simulink model "GA_NoSin_Lin"  (R2017a)
settings: Solver=FixedStepAuto  StartTime=0.0  StopTime=4*pi  MaxStep=1e-4  RelTol=1e-6
libraries: powerlib x6, powerlib_meascontrol x3
settings Model: Creator=pagilm  LastModifiedBy=pagilm

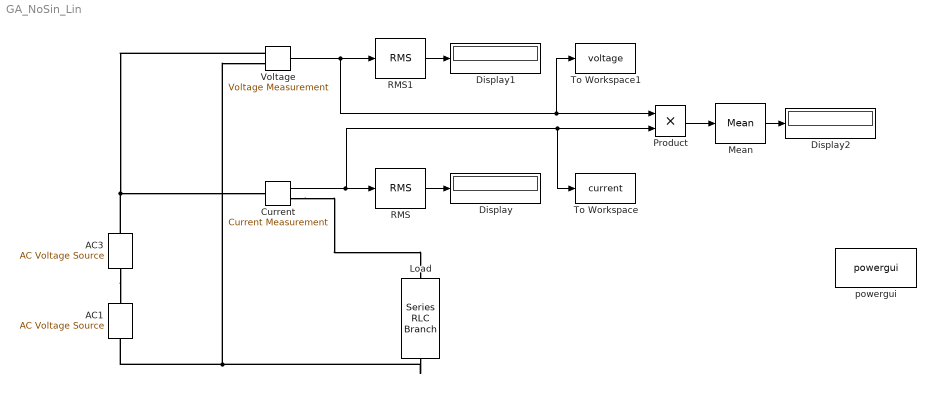
== system GA_NoSin_Lin ==
  AC1 : powerlib/Electrical Sources/AC Voltage Source  Amplitude=200*sqrt(2)  Phase=0  Frequency=1/2/pi  SampleTime=0  Measurements=None  BusType=swing  Pref=10e3  Qref=0  Qmin=-inf  Qmax=+inf
  AC3 : powerlib/Electrical Sources/AC Voltage Source  Amplitude=200*sqrt(2)  Phase=0  Frequency=3/2/pi  SampleTime=0  Measurements=None  BusType=swing  Pref=10e3  Qref=0  Qmin=-inf  Qmax=+inf
  "Current " : powerlib/Measurements/Current Measurement  PhasorSimulation=off  OutputType=Complex  PSBequivalent=0
  Display : Display
  Display1 : Display
  Display2 : Display
  Load : powerlib/Elements/Series RLC Branch  LConnTagsString=__new0  RConnTagsString=__new0  BranchType=RLC  Resistance=1  Inductance=3/4  SetiL0=off  InitialCurrent=0  Capacitance=4/15  Setx0=off  InitialVoltage=0  Measurements=None
  Mean : powerlib_meascontrol/Measurements/Mean  Freq=1/2/pi  Vinit=0  Ts=0
  Product : Product
  RMS : powerlib_meascontrol/Measurements/RMS  TrueRMS=on  Freq=1/2/pi  RMSInit=0  Ts=0
  RMS1 : powerlib_meascontrol/Measurements/RMS  TrueRMS=on  Freq=1/2/pi  RMSInit=0  Ts=0
  To Workspace : ToWorkspace  VariableName=current  SaveFormat=Structure With Time  SampleTime=-1
  To Workspace1 : ToWorkspace  VariableName=voltage  SaveFormat=Structure With Time  SampleTime=-1
  "Voltage " : powerlib/Measurements/Voltage Measurement  PhasorSimulation=off  OutputType=Complex  PSBequivalent=0
  powergui : powerlib/powergui  Priority=1  SimulationMode=Discrete  SampleTime=50e-6  frequency=60  Iterations=50  frequencyindice=0.159154943091895  Pbase=100e6  ErrMax=1e-4  UnitsV=kV  UnitsW=MW  buscounter=0  FunctionMessages=off  echomessages=off  EnableUseOfTLC=off  CurrentSourceSwitches=off  DisableSnubberDevices=off  DisableRonSwitches=off  DisableVfSwitches=off  DisplayEquations=off  SolverType=Tustin/Backward Euler (TBE)  Interpol=off  ExternalGateDelay=off  methode=off  Ts=100  x0status=blocks  SPID=off  SwTol=0  HookPort=off  RestoreLinks=warning  ResistiveCurrentMeasurement=off  Frange=[0:2:500]  Ylog=off  Xlog=on  ShowGrid=off  save=off  variable=ZData  structure=corriente  ZoomFFT=off  StartTime=0.0  cycles=1  DisplayStyle=1  fundamental=50  FreqAxis=on  MaxFrequency=1000  frequencyindicesteady=1  RmsSteady=1  display=off
  wires:
  "Current "/1 -> To Workspace/1, Product/2, RMS/1
  "Voltage "/1 -> To Workspace1/1, Product/1, RMS1/1
  RMS/1 -> Display/1
  RMS1/1 -> Display1/1
  Product/1 -> Mean/1
  Mean/1 -> Display2/1
  connections:
  "Voltage "/LConn1 -- "Current "/LConn1 -- AC3/RConn1
  "Current "/RConn1 -- Load/LConn1
  Load/RConn1 -- AC1/LConn1 -- "Voltage "/LConn2
  AC3/LConn1 -- AC1/RConn1
